simulink model "Interface_1"  (R2021a)
settings: Solver=VariableStepAuto  StartTime=0.0  StopTime=2000  RelTol=1e-3
libraries: audiosources x3, dspsnks4 x1, dspspect3 x1
settings Model: Creator=vpixx  LastModifiedBy=vpixx

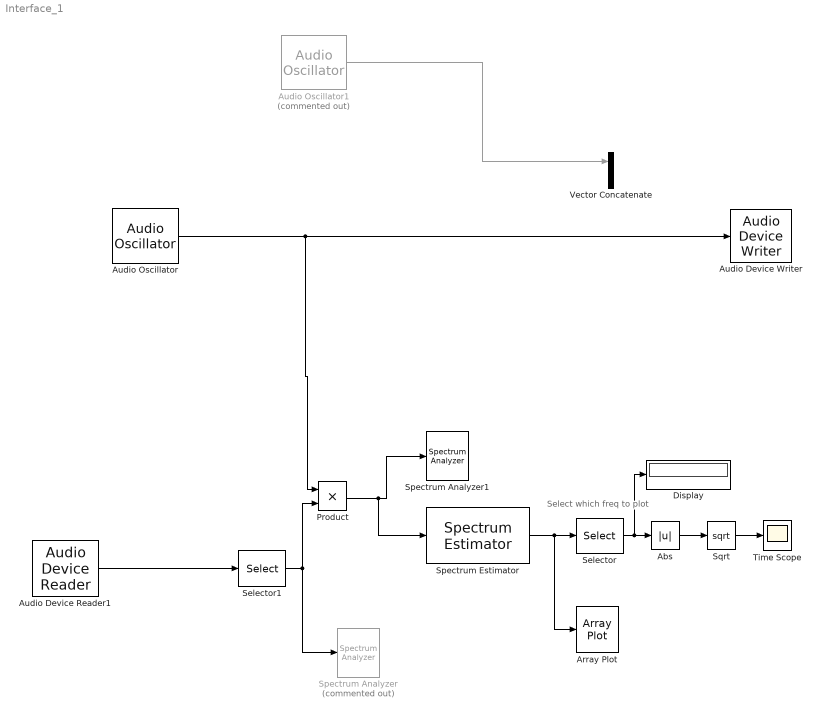
== system Interface_1 ==
  note: Select which freq to plot
  Abs : Abs
  Array Plot : ArrayPlot  WindowPosition=[-2482.000000,884.000000,1209.000000,747.000000,]  PlotType=Line  YLimits=[-157.80667772234602,-115.09657083278863]  DefaultConfigurationName=dsp.scopes.ArrayPlotBlockSpecification
  Audio Device Reader1 : audiosources/Audio Device Reader  Driver=ASIO  Device=M-Audio AIR 192 14 ASIO  SampleRate=192000  NumChannels=6  SamplesPerFrame=1024  BitDepth=24-bit integer  NumBuffers=10  DefaultInputChannelMapping=on  InputChannelMapping=1  OutputNumOverrunSamples=off  OutputDataType=double  DriverIdx=3  DeviceWarnFlag=''
      settings: SourceProductBaseCode=AU
  Audio Device Writer : dspsnks4/Audio Device Writer  Driver=ASIO  Device=M-Audio AIR 192 14 ASIO  InheritSampleRate=off  SampleRate=192000  BitDepth=24-bit integer  BufferSize=4096  NumBuffers=10  DefaultOutputChannelMapping=on  OutputChannelMapping=1  OutputNumUnderrunSamples=off  DriverIdx=3  DeviceWarnFlag=''
  Audio Oscillator : audiosources/Audio Oscillator  FrequencyPort=off  Frequency=15000  AmplitudePort=off  Amplitude=1  DCOffsetPort=off  PhaseOffset=0.25  DCOffset=0  WidthPort=off  Width=1  DutyCyclePort=off  DutyCycle=0.5  SampsPerFrame=1024  Fs=192000  OutputDataType=double  SimulateUsing=Code generation
      settings: SourceProductBaseCode=AU  SignalType=sine
  Audio Oscillator1 : audiosources/Audio Oscillator  Commented=on  FrequencyPort=off  Frequency=19000  AmplitudePort=off  Amplitude=1  DCOffsetPort=off  PhaseOffset=0  DCOffset=0  WidthPort=off  Width=1  DutyCyclePort=off  DutyCycle=0.5  SampsPerFrame=1024  Fs=192000  OutputDataType=double  SimulateUsing=Code generation
      settings: SourceProductBaseCode=AU  SignalType=sine
  Display : Display
  Product : Product
  Selector : Selector  NumberOfDimensions=2  IndexMode=Zero-based  InputPortWidth=3  IndexOptions=Index vector (dialog),Index vector (dialog)  Indices=0,0  OutputSizes=1,1
  Selector1 : Selector  NumberOfDimensions=2  InputPortWidth=3  IndexOptions=Index vector (dialog),Index vector (dialog)  Indices=1:1024,1  OutputSizes=1,1
  Spectrum Analyzer : SpectrumAnalyzer  Commented=on
  Spectrum Analyzer1 : SpectrumAnalyzer
  Spectrum Estimator : dspspect3/Spectrum Estimator  Method=Welch  NumTapsPerBand=2  SpectrumType=Power density  FrequencyResolutionMethod=Auto  FilterBankResolutionMethod=Auto  RBW=5  WindowLength=1024  FrequencyBandsSource=Same as input frame size  FrequencyBands=1024  FFTLengthSource=Auto  FFTLength=1024  InheritSampleRate=on  SampleRate=192000  Window=Hann  SidelobeAttenuation=60  AveragingMethod=Running  SpectralAverages=150  ForgettingFactorPort=off  ForgettingFactor=0.9  Overlap=0  ReferenceLoad=1000  FrequencyRange=One-sided  PowerUnits=dBm  OutputMaxHoldSpectrum=off  OutputMinHoldSpectrum=off  OutputFrequencyVector=off  OutputRBW=off  SimulateUsing=Code generation
      settings: SourceProductBaseCode=DS
  Sqrt : Sqrt  SaturateOnIntegerOverflow=on
  Time Scope : Scope
  Vector Concatenate : Concatenate  Mode=Multidimensional array  ConcatenateDimension=2
  wires:
  Audio Device Reader1/1 -> Selector1/1
  Product/1 -> Spectrum Estimator/1, Spectrum Analyzer1/1
  Spectrum Estimator/1 -> Array Plot/1, Selector/1
  Selector/1 -> Display/1, Abs/1
  Sqrt/1 -> Time Scope/1
  Abs/1 -> Sqrt/1
  Audio Oscillator/1 -> Product/1, Audio Device Writer/1
  Audio Oscillator1/1 -> Vector Concatenate/1
  Selector1/1 -> Product/2, Spectrum Analyzer/1
